simulink model "FlightGear_BUS_aerosurface"  (R2017a)
settings: Solver=VariableStepAuto  StartTime=0.0  StopTime=20  FixedStep=0.01  RelTol=1e-2
values from neighbouring files (symbols this model uses):
  a0_s2345 = [0;0;0.05;0.05]    [HW5_4_surfaces.m]    (also in TEST_aerosetup.m; surfaces_setup_test.m)
  A_2345 = c_2345.*b_2345    [HW5_4_surfaces.m]    (also in TEST_aerosetup.m; surfaces_setup_test.m)
  Aileron_left = 0    [HW5_4_surfaces.m]    (also in TEST_aerosetup.m; surfaces_setup_test.m)
  Aileron_right = 0    [HW5_4_surfaces.m]    (also in TEST_aerosetup.m; surfaces_setup_test.m)
  c_2345 = [0.075;0.08;0.1;0.1]    [HW5_4_surfaces.m]    (also in TEST_aerosetup.m; surfaces_setup_test.m)
  CD0_s2345 = [0.01;0.01;0.01;0.01]    [HW5_4_surfaces.m]    (also in TEST_aerosetup.m; surfaces_setup_test.m)
  CDa_s2345 = [1;1;1;1]    [HW5_4_surfaces.m]    (also in TEST_aerosetup.m; surfaces_setup_test.m)
  CL0_2345 = [0;0; 0.05; 0.05]    [HW5_4_surfaces.m]    (also in TEST_aerosetup.m; surfaces_setup_test.m)
  CLa = 2*pi*(r./(2+r))    [HW5_4_surfaces.m]    (also in TEST_aerosetup.m; surfaces_setup_test.m)
  CM0_s2345 = [0;0;-0.05;-0.05]    [HW5_4_surfaces.m]    (also in TEST_aerosetup.m; surfaces_setup_test.m)
  CMa_s2345 = [0; 0; 0; 0]    [HW5_4_surfaces.m]    (also in TEST_aerosetup.m; surfaces_setup_test.m)
  e_s2345 = [0.8;0.8;0.9;0.9]    [HW5_4_surfaces.m]    (also in TEST_aerosetup.m; surfaces_setup_test.m)
  elevator = 0    [HW5_4_surfaces.m]    (also in TEST_aerosetup.m; surfaces_setup_test.m)
  Fext_N = -g_EN * m    [HW5_4_surfaces.m]    (also in TEST_aerosetup.m = [10 10 10]; surfaces_setup_test.m)
  g_EN = [0; 0; 9.81]    [HW5_4_surfaces.m]    (also in TEST_aerosetup.m = [0; 0; 9.8]; surfaces_setup_test.m)
  i_s2345 = [0; 0; 0.05; 0.05;]    [HW5_4_surfaces.m]    (also in TEST_aerosetup.m; surfaces_setup_test.m)
  J_cgp = ones(3)    [surfaces_setup_test.m]
  M_total = sum(MnG(:,1))/1000    [HW5_4_surfaces.m]    (also in TEST_aerosetup.m; surfaces_setup_test.m = sum(MnG1(:,1))/1000)
  Mext_B = [0; 0; 0]    [HW5_4_surfaces.m]    (also in TEST_aerosetup.m = [1; 1; 1]; surfaces_setup_test.m)
  p_E_BE_ini = p_E_BE_ini_deg .* [deg2rad; deg2rad; 1]    [HW5_4_surfaces.m]    (also in TEST_aerosetup.m; surfaces_setup_test.m)
  r = b_2345./c_2345    [HW5_4_surfaces.m]    (also in TEST_aerosetup.m; surfaces_setup_test.m)
  Rearth = 6371000    [HW5_4_surfaces.m]    (also in TEST_aerosetup.m; surfaces_setup_test.m)
  rudder = 0    [HW5_4_surfaces.m]    (also in TEST_aerosetup.m; surfaces_setup_test.m)
  Theta_ini = Theta_ini_deg * deg2rad    [HW5_4_surfaces.m]    (also in TEST_aerosetup.m; surfaces_setup_test.m)
  v_N_AE = [0;0;0]    [HW5_4_surfaces.m]    (also in TEST_aerosetup.m; surfaces_setup_test.m)
  Vbbe_int = [10; 0; 0]    [HW5_4_surfaces.m]    (also in TEST_aerosetup.m; surfaces_setup_test.m = [5; 0; 0])
  w_B_BE_ini = [1e0; 1e-2; 1e-2]    [HW5_4_surfaces.m]    (also in TEST_aerosetup.m; surfaces_setup_test.m)
  xyz_s = [[-0.76 0 0.16];[-0.76 0 -0.09];[-0.23 0.44 0];[-0.23 -0.44 0];]    [HW5_4_surfaces.m]    (also in TEST_aerosetup.m; surfaces_setup_test.m)
undefined symbols (not defined in the file or in its folder): Earth, J_propeller, WGS84
libraries: dspinverses x6, vrlib x5, simulink x4, sharedtransform x2, aerolibtransform2 x2, aerolibfltsims x2, aerolibutil x2, sharedutil x2, commrandsrc3 x1
(part 2 of 2)

== matlab function FlightGear_BUS_aerosurface/with propeller/AeroSurface controller/MATLAB Function ==
  data: V_B_BA input; V_inf input; F_b output; alp input; bet input; M_b output; CLa parameter; i_s2345 parameter; CL0_2345 parameter; a0_s2345 parameter; e_s2345 parameter; CDa_s2345 parameter; CD0_s2345 parameter; CM0_s2345 parameter; A_2345 parameter; xyz_s parameter; r parameter; CMa_s2345 parameter; c_2345 parameter; aileron_r input; aileron_l input; elevator input; rudder input
function [F_b, M_b] = fcn(V_B_BA,V_inf, alp,bet, CLa, i_s2345, CL0_2345, a0_s2345, e_s2345, CDa_s2345, CD0_s2345, CM0_s2345, A_2345, xyz_s, r, CMa_s2345, c_2345, aileron_r, aileron_l, elevator, rudder)
%% Properties
% CLa=2*pi*(r./(2+r)); 
% % V_B_BA=[ 1 1 1];V_inf=norm(V_B_BA); 
V_B_BA_0=[ V_B_BA(1); V_B_BA(2); V_B_BA(3)];
n1=[0,0,-1]; n2=[0,1,0]; n3=[0,0,-1]; n4=[0,0,-1]; 


a_ss1=i_s2345(1)-asin(complex(V_B_BA_0*n1)/V_inf);
a_ss2=i_s2345(2)-asin(complex(V_B_BA_0*n2)/V_inf);
a_ss3=i_s2345(3)-asin(complex(V_B_BA_0*n3)/V_inf);
a_ss4=i_s2345(4)-asin(complex(V_B_BA_0*n4)/V_inf);

a1=a_ss1-a0_s2345(1);
a2=a_ss2-a0_s2345(2);
a3=a_ss3-a0_s2345(3);
a4=a_ss4-a0_s2345(4);
%% for lift
CL1=CL0_2345(1)+CLa(1).*a_ss1+3*elevator*0.5;   %(0.075*0.35*0.2)/0.075*0.35; full span control surface
CL2=CL0_2345(2)+CLa(2).*a_ss2+3*rudder*0.5;   %(0.08*0.08*0.2)/(0.08*0.08); %Apply to fulsage(x*z) 
CL3=CL0_2345(3)+CLa(3).*a_ss3+3*aileron_r*0.5; %(0.02*0.96)/(0.1*0.96); 
CL4=CL0_2345(4)+CLa(4).*a_ss4+3*aileron_l*0.5;  %(0.02*0.96)/(0.1*0.96); %servo/wing

L1= CL1.*A_2345(1)*(0.5*(V_inf^2));
L2= CL2.*A_2345(2)*(0.5*(V_inf^2));
L3= CL3.*A_2345(3)*(0.5*(V_inf^2));
L4= CL4.*A_2345(4)*(0.5*(V_inf^2));


%% For Drag
cdl1=CL1.^2./(pi*(e_s2345(1).*r(1))); 
cdl2=CL2.^2./(pi*(e_s2345(2).*r(2))); 
cdl3=CL3.^2./(pi*(e_s2345(3).*r(3))); 
cdl4=CL4.^2./(pi*(e_s2345(4).*r(4)));

CD1=CD0_s2345(1)+CDa_s2345(1).*(a1.*a1)+cdl1;
CD2=CD0_s2345(2)+CDa_s2345(2).*(a2.*a2)+cdl2;
CD3=CD0_s2345(3)+CDa_s2345(3).*(a3.*a3)+cdl3;
CD4=CD0_s2345(4)+CDa_s2345(4).*(a4.*a4)+cdl4;

D1=CD1.*A_2345(1)*(0.5*V_inf.^2);
D2=CD2.*A_2345(2)*(0.5*V_inf.^2);
D3=CD3.*A_2345(3)*(0.5*V_inf.^2);
D4=CD4.*A_2345(4)*(0.5*V_inf.^2);
%% For moment
CM1=CM0_s2345(1)+CMa_s2345(1).*a_ss1;
CM2=CM0_s2345(2)+CMa_s2345(2).*a_ss2;
CM3=CM0_s2345(3)+CMa_s2345(3).*a_ss3;
CM4=CM0_s2345(4)+CMa_s2345(4).*a_ss4;
M1=CM1.*A_2345(1).*c_2345(1)*(0.5*V_inf.^2);
M2=CM2.*A_2345(2).*c_2345(2)*(0.5*V_inf.^2);
M3=CM3.*A_2345(3).*c_2345(3)*(0.5*V_inf.^2);
M4=CM4.*A_2345(4).*c_2345(4)*(0.5*V_inf.^2);

%% for fulsage
CD_f=0.5; %%% from 0.5 to 1
D_fulsage=CD_f.*0.001*(0.5*V_inf.^2);
F_fulsage=-[D_fulsage;0;0];

%% For F_b inner
n11=[0;0;-1]; n22=[0;1;0]; n33=[0;0;-1]; n44=[0;0;-1]; 
F_surf1=L1*n11-[norm(D1);0;0];
F_surf2=L2*n22-[norm(D2);0;0];
F_surf3=L3*n33-[norm(D3);0;0];
F_surf4=L4*n44-[norm(D4);0;0];

Csb=[cos(alp), 0, sin(alp); 0, 1,0; -1*sin(alp) 0 cos(alp)];
Cws=[cos(bet),sin(bet),0 ; -1*sin(bet),cos(bet),0;0, 0 ,1];
Cwb=Cws*Csb;
Cbw=inv(Cwb);


F_b1=Cbw*F_surf1;F_b2=Cbw*F_surf2;F_b3=Cbw*F_surf3;F_b4=Cbw*F_surf4;F_b5=Cbw*F_fulsage;
% F_surf=F_surf1+F_surf2+F_surf3+F_surf4+F_fulsage;

F_b=F_b1+F_b2+F_b3+F_b4+F_b5;

% c=cross(xyz_s(i,:),F_b(:,1));
C=[0,0,0;0,0,-1;0, 1,0];
% M_s2345=zeros(3,4);
T1=transpose(cross(xyz_s(1,:),F_b1));
T2=transpose(cross(xyz_s(2,:),F_b2));
T3=transpose(cross(xyz_s(3,:),F_b3));
T4=transpose(cross(xyz_s(4,:),F_b4));
M_b1=M1*C*n11+T1;
M_b2=M2*C*n22+T2;
M_b3=M3*C*n33+T3;
M_b4=M4*C*n44+T4;
M_b=M_b1+M_b2+M_b3+M_b4;
end

== matlab function FlightGear_BUS_aerosurface/Rot kine/Euler to Quat  ==
  data: att input; H output
function H = fcn(att)
%#codegen
phi=att(1);
theta=att(2);
%psi=theta(3); %not needed for Euler Rotational Kinematics Matrix
H=[1,tan(theta)*sin(phi),tan(theta)*cos(phi); 0,cos(phi),-sin(phi);0,sin(phi)/cos(theta),cos(phi)/cos(theta)];

== matlab function FlightGear_BUS_aerosurface/with propeller/Rot kine/Euler to Quat  ==
  data: att input; H output
function H = fcn(att)
%#codegen
phi=att(1);
theta=att(2);
%psi=theta(3); %not needed for Euler Rotational Kinematics Matrix
H=[1,tan(theta)*sin(phi),tan(theta)*cos(phi); 0,cos(phi),-sin(phi);0,sin(phi)/cos(theta),cos(phi)/cos(theta)];

== matlab function FlightGear_BUS_aerosurface/Rot kine/Quat2Euler 1 ==
  data: Q input; theta output
function theta = fcn(Q)
q0=Q(1);
q1=Q(2);
q2=Q(3);
q3=Q(4);
roll=atan2(2*(q0*q1+q2*q3),q0^2-q1^2-q2^2+q3^2); 
pitch=asin(2*(q0*q2-q1*q3)); 
yaw=atan2(2*(q0*q3+q1*q2),q0^2+q1^2-q2^2-q3^2);
theta=[roll;pitch;yaw];

== matlab function FlightGear_BUS_aerosurface/Rot kine/Euler to Quat 3 ==
  data: att input; Q output
function Q = fcn(att)
phi=att(1);
theta=att(2);
psi=att(3);
q0=cos(phi/2)*cos(theta/2)*cos(psi/2)+sin(phi/2)*sin(theta/2)*sin(psi/2); 
q1=sin(phi/2)*cos(theta/2)*cos(psi/2)-cos(phi/2)*sin(theta/2)*sin(psi/2); 
q2=cos(phi/2)*sin(theta/2)*cos(psi/2)+sin(phi/2)*cos(theta/2)*sin(psi/2); 
q3=cos(phi/2)*cos(theta/2)*sin(psi/2)-sin(phi/2)*sin(theta/2)*cos(psi/2);
Q=[q0;q1;q2;q3];

== matlab function FlightGear_BUS_aerosurface/with propeller/Rot kine/Euler to Quat 1 ==
  data: att input; H output
function H = fcn(att)
%#codegen
phi=att(1);
theta=att(2);
%psi=theta(3); %not needed for Euler Rotational Kinematics Matrix
H=[1,tan(theta)*sin(phi),tan(theta)*cos(phi); 0,cos(phi),-sin(phi);0,sin(phi)/cos(theta),cos(phi)/cos(theta)];

== matlab function FlightGear_BUS_aerosurface/with propeller/Rot kine/Euler to Quat 3 ==
  data: att input; Q output
function Q = fcn(att)
phi=att(1);
theta=att(2);
psi=att(3);
q0=cos(phi/2)*cos(theta/2)*cos(psi/2)+sin(phi/2)*sin(theta/2)*sin(psi/2); 
q1=sin(phi/2)*cos(theta/2)*cos(psi/2)-cos(phi/2)*sin(theta/2)*sin(psi/2); 
q2=cos(phi/2)*sin(theta/2)*cos(psi/2)+sin(phi/2)*cos(theta/2)*sin(psi/2); 
q3=cos(phi/2)*cos(theta/2)*sin(psi/2)-sin(phi/2)*sin(theta/2)*cos(psi/2);
Q=[q0;q1;q2;q3];

== matlab function FlightGear_BUS_aerosurface/with propeller/Rot kine/Quat2Euler 1 ==
  data: Q input; theta output
function theta = fcn(Q)
q0=Q(1);
q1=Q(2);
q2=Q(3);
q3=Q(4);
roll=atan2(2*(q0*q1+q2*q3),q0^2-q1^2-q2^2+q3^2); 
pitch=asin(2*(q0*q2-q1*q3)); 
yaw=atan2(2*(q0*q3+q1*q2),q0^2+q1^2-q2^2-q3^2);
theta=[roll;pitch;yaw];

== matlab function FlightGear_BUS_aerosurface/with propeller/new tran kine sph/p2Cne/LAT DCM ==
  data: u input; y output
function y = fcn(u)
y = [cos(u) 0 sin(u); 0 1 0; -sin(u) 0 cos(u)];

== matlab function FlightGear_BUS_aerosurface/new tran kine sph/sph_trans ==
  data: P_BE_E_ini input; X_BE_E_ini output
function X_BE_E_ini = fcn(P_BE_E_ini)
lat=P_BE_E_ini(1);
lon=P_BE_E_ini(2);
alt=P_BE_E_ini(3);
a = 6378000;
e = 8.1819190842622e-2;
N = a ./ sqrt(1 - e^2 .* sin(lat).^2);
x = (N+alt) .* cos(lat) .* cos(lon);
y = (N+alt) .* cos(lat) .* sin(lon);
z = ((1-e^2) .* N + alt) .* sin(lat);
X_BE_E_ini=[(N+alt) .* cos(lat) .* cos(lon); (N+alt) .* cos(lat) .* sin(lon);((1-e^2) .* N + alt) .* sin(lat)];

== matlab function FlightGear_BUS_aerosurface/with propeller/new tran kine sph/p2Cne/LON DCM ==
  data: u input; y output
function y = fcn(u)

y = [1, 0, 0;0, cos(u), sin(u);0, -sin(u), cos(u)];

== matlab function FlightGear_BUS_aerosurface/with propeller/new tran kine sph/sph_trans ==
  data: P_BE_E_ini input; X_BE_E_ini output
function X_BE_E_ini = fcn(P_BE_E_ini)
lat=P_BE_E_ini(1);
lon=P_BE_E_ini(2);
alt=P_BE_E_ini(3);
a = 6378000;
e = 8.1819190842622e-2;
N = a ./ sqrt(1 - e^2 .* sin(lat).^2);
x = (N+alt) .* cos(lat) .* cos(lon);
y = (N+alt) .* cos(lat) .* sin(lon);
z = ((1-e^2) .* N + alt) .* sin(lat);
X_BE_E_ini=[(N+alt) .* cos(lat) .* cos(lon); (N+alt) .* cos(lat) .* sin(lon);((1-e^2) .* N + alt) .* sin(lat)];

== matlab function FlightGear_BUS_aerosurface/with propeller/Rot dyn1/Subsystem/3*3 ome matrix ==
  data: u input; y output
function y = fcn(u)
p=u(1);
q=u(2);
r=u(3);
y=[ 0, -r q;r 0 -p; -q p 0];
